simulink model "Multi_agent_MIMO"  (R2022b)
settings: Solver=VariableStepAuto  StartTime=0.0  StopTime=10.0  RelTol=1e-3
undefined symbols (not defined in the file): Angular, Linear
libraries: robotlib x9
settings Model: Creator=yoav  LastModifiedBy=yoav

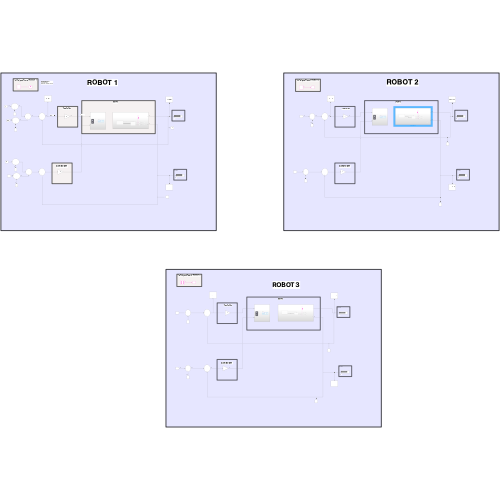
[thumbnail: Simulink's stored preview of the top-level diagram]
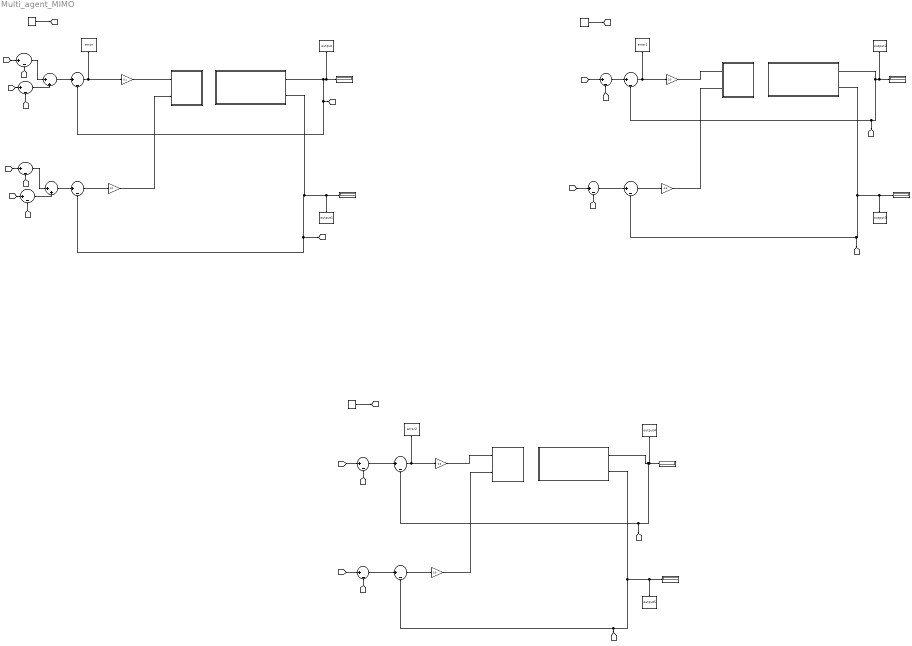
== system Multi_agent_MIMO ==
  note: The user need to
      |  put the initial position
      |  of the robot as it
      |  apperas in the spawn service
  note: $V_{command}(t)$
  note: Error - $e(t)$
  note: X
  note: Position
  note: ROBOT 2
  note: Controller
  note: Controller
  note: Controller
  note: Y
  note: Plant
  note: Position
  note: Plant
  note: Position
  note: X
  note: Controller
  note: Y
  note: Position
  note: Y
  note: Controller
  note: Position
  note: Plant
  note: X
  note: Position
  note: Controller
  note: ROBOT 1
  note: ROBOT 3
  note: Initial position of ROBOT 1
  note: Initial position of ROBOT 2
  note: Initial position of ROBOT 3
  Constant1 : Constant  Value="[5 ;  8]"  VectorParams1D=off
  Constant2 : Constant  Value="[2 ;  -4]"  VectorParams1D=off
  Constant6 : Constant  Value="[-6 ;  2]"  VectorParams1D=off
  Display{1..6} (6 alike) : Display
  Gain1 : Gain  Gain=0.1
  Gain2 : Gain  Gain=0.1
  Gain{3..6} (4 alike) : Gain  Gain=0.5
  Subsystem : Subsystem
  Subsystem1 : Subsystem
  Subsystem2 : Subsystem
  Subsystem3 : Subsystem
  Subsystem4 : Subsystem
  Subsystem5 : Subsystem
  Sum{,1..5,7..8,10..15} (14 alike) : Sum  Inputs=|+-
  Sum6 : Sum  Inputs=|++
  Sum9 : Sum  Inputs=|++
  To Workspace : ToWorkspace  VariableName=error  SaveFormat=Timeseries  SampleTime=-1
  To Workspace1 : ToWorkspace  VariableName=output  SaveFormat=Timeseries  SampleTime=-1
  To Workspace2 : ToWorkspace  VariableName=output1  SaveFormat=Timeseries  SampleTime=-1
  To Workspace3 : ToWorkspace  VariableName=error1  SaveFormat=Timeseries  SampleTime=-1
  To Workspace4 : ToWorkspace  VariableName=output2  SaveFormat=Timeseries  SampleTime=-1
  To Workspace5 : ToWorkspace  VariableName=output3  SaveFormat=Timeseries  SampleTime=-1
  To Workspace6 : ToWorkspace  VariableName=error2  SaveFormat=Timeseries  SampleTime=-1
  To Workspace7 : ToWorkspace  VariableName=output4  SaveFormat=Timeseries  SampleTime=-1
  To Workspace8 : ToWorkspace  VariableName=output5  SaveFormat=Timeseries  SampleTime=-1
  tag scope: IC1=global, IC2=global, IC3=global
  wires:
  Sum12/1 -> Sum2/1
  [Y2] -> Sum13/2
  Subsystem1/1(Output) -> Sum/2, [X1], Display3/1, To Workspace1/1
  [Y1] -> Sum10/2
  Sum5/1 -> Gain6/1
  [X3] -> Sum14/2
  Gain4/1 -> Subsystem2/2(In2)
  Gain5/1 -> Subsystem4/1(In1)
  Subsystem3/1(Output) -> [X2], Sum2/2, Display4/1, To Workspace4/1
  [X1] -> Sum14/1
  [Y1] -> Sum15/1
  Sum7/1 -> Sum6/1
  Sum9/1 -> Sum1/1
  Sum8/1 -> Sum6/2
  Sum14/1 -> Sum4/1
  Sum10/1 -> Sum9/1
  [X2] -> Sum12/2
  [Y3] -> Sum15/2
  Gain2/1 -> Subsystem/2(In2)
  Sum/1 -> To Workspace/1, Gain1/1
  Sum6/1 -> Sum/1
  Subsystem1/2(Out1) -> Sum1/2, [Y1], Display1/1, To Workspace2/1
  Subsystem3/2(Out1) -> [Y2], Sum3/2, Display2/1, To Workspace5/1
  [Y1] -> Sum11/2
  [Y2] -> Sum10/1
  Sum1/1 -> Gain2/1
  Gain3/1 -> Subsystem2/1(In1)
  [X2] -> Sum7/1
  Sum2/1 -> To Workspace3/1, Gain3/1
  Sum13/1 -> Sum3/1
  Sum15/1 -> Sum5/1
  Sum3/1 -> Gain4/1
  Sum4/1 -> To Workspace6/1, Gain5/1
  Sum11/1 -> Sum9/2
  Gain6/1 -> Subsystem4/2(In2)
  [X1] -> Sum12/1
  [X1] -> Sum7/2
  [X3] -> Sum8/1
  [Y3] -> Sum11/1
  Subsystem5/2(Out1) -> Sum5/2, [Y3], Display5/1, To Workspace8/1
  [X1] -> Sum8/2
  Subsystem5/1(Output) -> Sum4/2, [X3], Display6/1, To Workspace7/1
  Gain1/1 -> Subsystem/1(In1)
  [Y1] -> Sum13/1
  Constant6/1 -> [IC1]
  Constant1/1 -> [IC2]
  Constant2/1 -> [IC3]

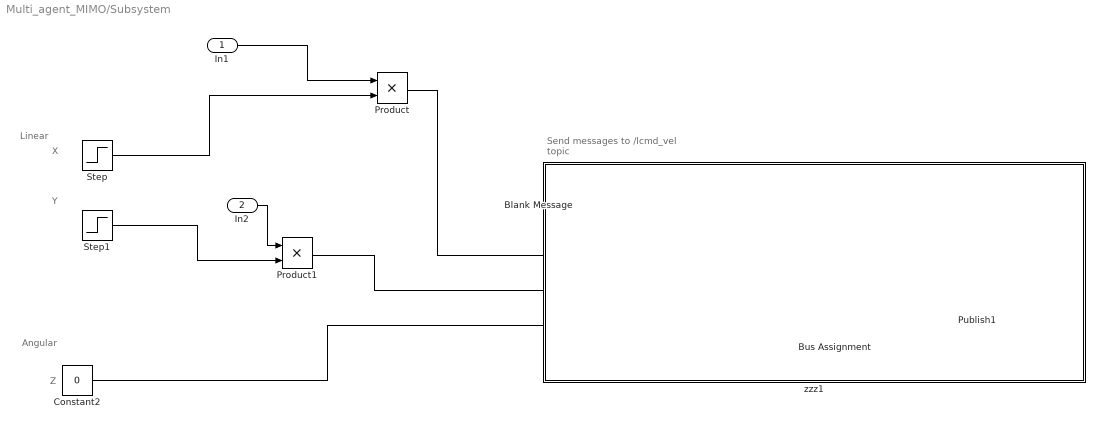
== system Multi_agent_MIMO/Subsystem ==
  note: Send messages to /lcmd_vel topic
  note: Y
  note: X
  note: Linear
  note: Angular
  note: Z
  In1 : Inport
  In2 : Inport  Port=2
  Blank Message : robotlib/Blank Message  messageClass=Message  entityType=geometry_msgs/Twist  messageType=geometry_msgs/Twist  SampleTime=inf  legacyBusStruct=off
  Bus Assignment : BusAssignment  AssignedSignals=Linear.X,Linear.Y,Angular.Z
  Constant2 : Constant  Value=0
  Product : Product
  Product1 : Product
  Publish1 : robotlib/Publish  topicSource=Specify your own  topic=/robot1/cmd_vel  messageType=geometry_msgs/Twist  legacyBusStruct=off  messageQueueLength=105
  Step : Step  Time=0  SampleTime=0
  Step1 : Step  Time=0  SampleTime=0
  zzz1 : Subsystem  TreatAsAtomicUnit=on
      settings: OpenFcn=% no-op
      mask Display: disp('')
  wires:
  Blank Message/1 -> Bus Assignment/1
  Bus Assignment/1 -> Publish1/1
  Constant2/1 -> Bus Assignment/4
  In1/1 -> Product/1
  Step/1 -> Product/2
  Product/1 -> Bus Assignment/2
  Step1/1 -> Product1/2
  In2/1 -> Product1/1
  Product1/1 -> Bus Assignment/3

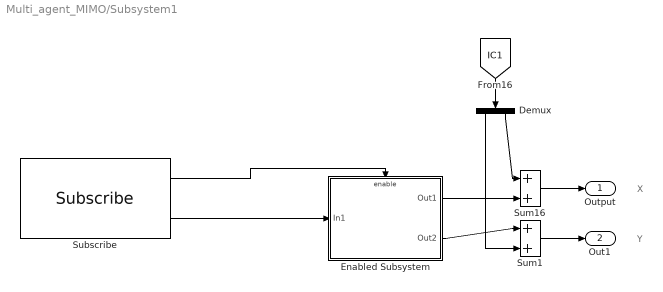
== system Multi_agent_MIMO/Subsystem1 ==
  note: X
  note: Y
  Demux : Demux  Outputs=2
  Enabled Subsystem : Subsystem  TreatAsAtomicUnit=on
  Subscribe : robotlib/Subscribe  topicSource=Select from ROS network  topic=/robot1/odom  messageType=nav_msgs/Odometry  SampleTime=-1  legacyBusStruct=off  messageQueueLength=1
      settings: LibrarySourceBlock=roslib/ROS/Subscribe
  Sum1 : Sum  Inputs=|++
  Sum16 : Sum  Inputs=|++
  Output : Outport
  Out1 : Outport  Port=2
  wires:
  Subscribe/2 -> Enabled Subsystem/1(In1)
  Subscribe/1 -> Enabled Subsystem/Enable
  Enabled Subsystem/1(Out1) -> Sum16/2
  [IC1] -> Demux/1
  Demux/2 -> Sum16/1
  Sum16/1 -> Output/1
  Enabled Subsystem/2(Out2) -> Sum1/1
  Demux/1 -> Sum1/2
  Sum1/1 -> Out1/1

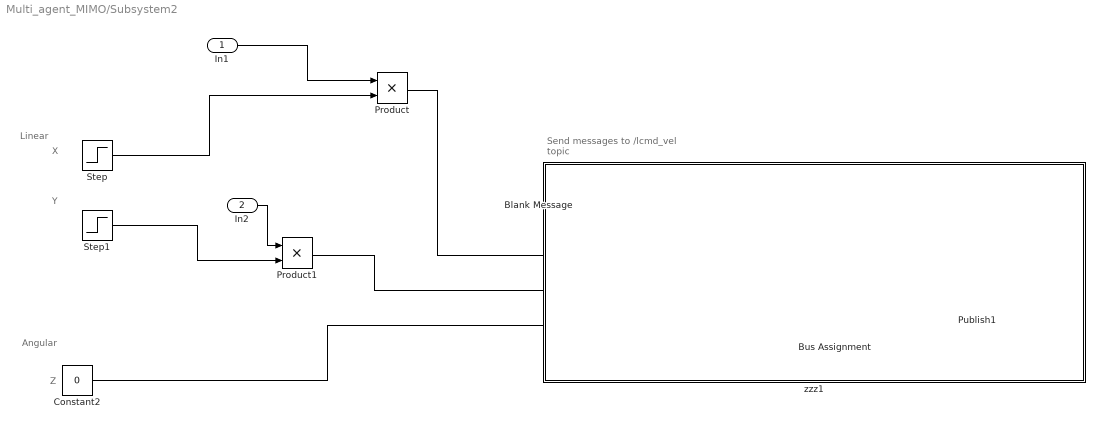
== system Multi_agent_MIMO/Subsystem2 ==
  note: Send messages to /lcmd_vel topic
  note: Y
  note: X
  note: Linear
  note: Angular
  note: Z
  In1 : Inport
  In2 : Inport  Port=2
  Blank Message : robotlib/Blank Message  messageClass=Message  entityType=geometry_msgs/Twist  messageType=geometry_msgs/Twist  SampleTime=inf  legacyBusStruct=off
  Bus Assignment : BusAssignment  AssignedSignals=Linear.X,Linear.Y,Angular.Z
  Constant2 : Constant  Value=0
  Product : Product
  Product1 : Product
  Publish1 : robotlib/Publish  topicSource=Specify your own  topic=/robot2/cmd_vel  messageType=geometry_msgs/Twist  legacyBusStruct=off  messageQueueLength=105
  Step : Step  Time=0  SampleTime=0
  Step1 : Step  Time=0  SampleTime=0
  zzz1 : Subsystem  TreatAsAtomicUnit=on
      settings: OpenFcn=% no-op
      mask Display: disp('')
  wires:
  Blank Message/1 -> Bus Assignment/1
  Bus Assignment/1 -> Publish1/1
  Constant2/1 -> Bus Assignment/4
  In1/1 -> Product/1
  Step/1 -> Product/2
  Product/1 -> Bus Assignment/2
  Step1/1 -> Product1/2
  In2/1 -> Product1/1
  Product1/1 -> Bus Assignment/3

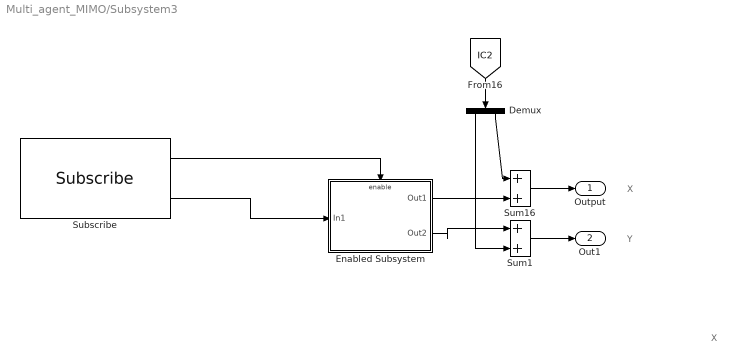
== system Multi_agent_MIMO/Subsystem3 ==
  note: X
  note: Y
  note: X
  Demux : Demux  Outputs=2
  Enabled Subsystem : Subsystem  TreatAsAtomicUnit=on
  Subscribe : robotlib/Subscribe  topicSource=Select from ROS network  topic=/robot2/odom  messageType=nav_msgs/Odometry  SampleTime=-1  legacyBusStruct=off  messageQueueLength=1
      settings: LibrarySourceBlock=roslib/ROS/Subscribe
  Sum1 : Sum  Inputs=|++
  Sum16 : Sum  Inputs=|++
  Output : Outport
  Out1 : Outport  Port=2
  wires:
  Subscribe/2 -> Enabled Subsystem/1(In1)
  Subscribe/1 -> Enabled Subsystem/Enable
  Enabled Subsystem/2(Out2) -> Sum1/1
  Demux/2 -> Sum16/1
  Enabled Subsystem/1(Out1) -> Sum16/2
  Demux/1 -> Sum1/2
  Sum1/1 -> Out1/1
  Sum16/1 -> Output/1
  [IC2] -> Demux/1

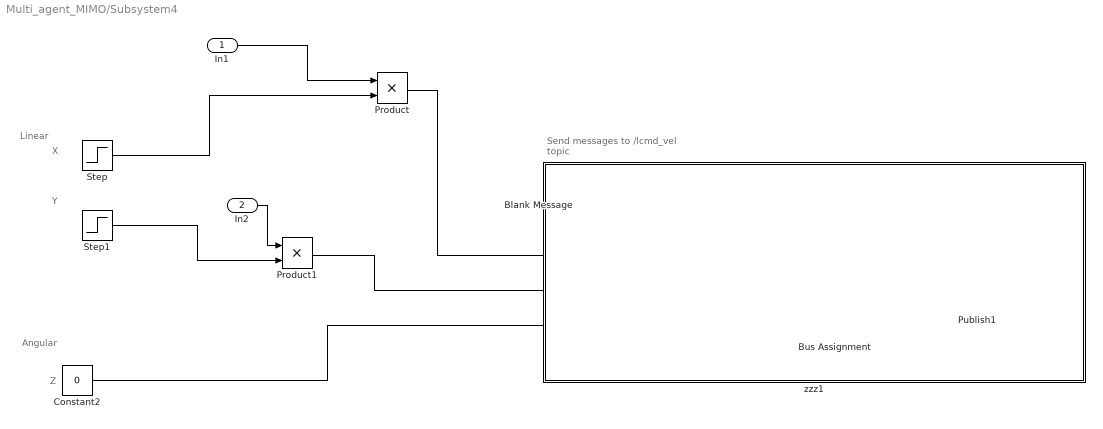
== system Multi_agent_MIMO/Subsystem4 ==
  note: Send messages to /lcmd_vel topic
  note: Y
  note: X
  note: Linear
  note: Angular
  note: Z
  In1 : Inport
  In2 : Inport  Port=2
  Blank Message : robotlib/Blank Message  messageClass=Message  entityType=geometry_msgs/Twist  messageType=geometry_msgs/Twist  SampleTime=inf  legacyBusStruct=off
  Bus Assignment : BusAssignment  AssignedSignals=Linear.X,Linear.Y,Angular.Z
  Constant2 : Constant  Value=0
  Product : Product
  Product1 : Product
  Publish1 : robotlib/Publish  topicSource=Specify your own  topic=/robot3/cmd_vel  messageType=geometry_msgs/Twist  legacyBusStruct=off  messageQueueLength=105
  Step : Step  Time=0  SampleTime=0
  Step1 : Step  Time=0  SampleTime=0
  zzz1 : Subsystem  TreatAsAtomicUnit=on
      settings: OpenFcn=% no-op
      mask Display: disp('')
  wires:
  Blank Message/1 -> Bus Assignment/1
  Bus Assignment/1 -> Publish1/1
  Constant2/1 -> Bus Assignment/4
  In1/1 -> Product/1
  Step/1 -> Product/2
  Product/1 -> Bus Assignment/2
  Step1/1 -> Product1/2
  In2/1 -> Product1/1
  Product1/1 -> Bus Assignment/3

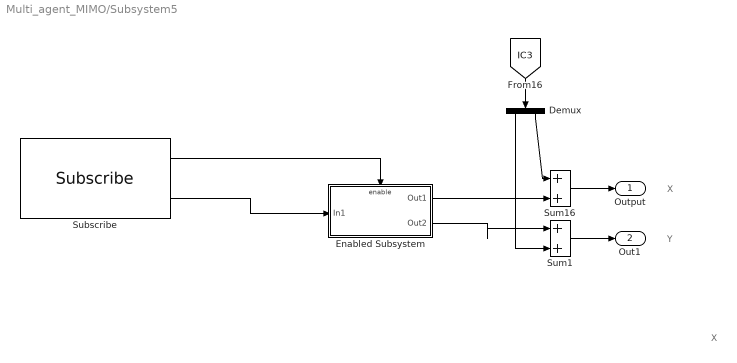
== system Multi_agent_MIMO/Subsystem5 ==
  note: X
  note: X
  note: Y
  Demux : Demux  Outputs=2
  Enabled Subsystem : Subsystem  TreatAsAtomicUnit=on
  Subscribe : robotlib/Subscribe  topicSource=Select from ROS network  topic=/robot3/odom  messageType=nav_msgs/Odometry  SampleTime=-1  legacyBusStruct=off  messageQueueLength=1
      settings: LibrarySourceBlock=roslib/ROS/Subscribe
  Sum1 : Sum  Inputs=|++
  Sum16 : Sum  Inputs=|++
  Output : Outport
  Out1 : Outport  Port=2
  wires:
  Subscribe/2 -> Enabled Subsystem/1(In1)
  Subscribe/1 -> Enabled Subsystem/Enable
  Enabled Subsystem/1(Out1) -> Sum16/2
  [IC3] -> Demux/1
  Sum16/1 -> Output/1
  Demux/1 -> Sum1/2
  Demux/2 -> Sum16/1
  Sum1/1 -> Out1/1
  Enabled Subsystem/2(Out2) -> Sum1/1

== system Multi_agent_MIMO/Subsystem/zzz1 ==

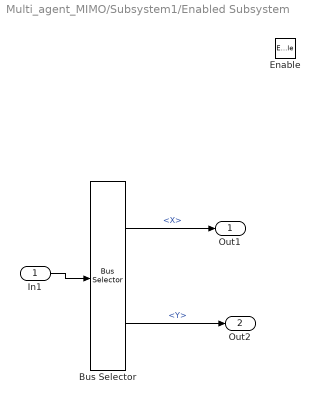
== system Multi_agent_MIMO/Subsystem1/Enabled Subsystem ==
  In1 : Inport
  Enable : EnablePort
  Bus Selector : BusSelector  OutputSignals=Pose.Pose.Position.X,Pose.Pose.Position.Y
  Out1 : Outport
  Out2 : Outport  Port=2
  wires:
  In1/1 -> Bus Selector/1
  Bus Selector/1 -> Out1/1  "<X>"
  Bus Selector/2 -> Out2/1  "<Y>"

== system Multi_agent_MIMO/Subsystem2/zzz1 ==

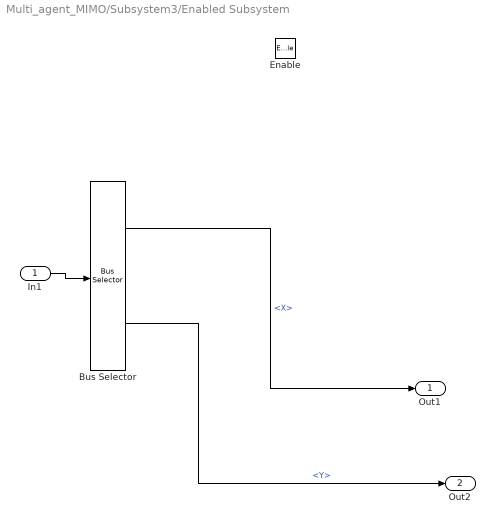
== system Multi_agent_MIMO/Subsystem3/Enabled Subsystem ==
  In1 : Inport
  Enable : EnablePort
  Bus Selector : BusSelector  OutputSignals=Pose.Pose.Position.X,Pose.Pose.Position.Y
  Out1 : Outport
  Out2 : Outport  Port=2
  wires:
  In1/1 -> Bus Selector/1
  Bus Selector/1 -> Out1/1  "<X>"
  Bus Selector/2 -> Out2/1  "<Y>"

== system Multi_agent_MIMO/Subsystem4/zzz1 ==

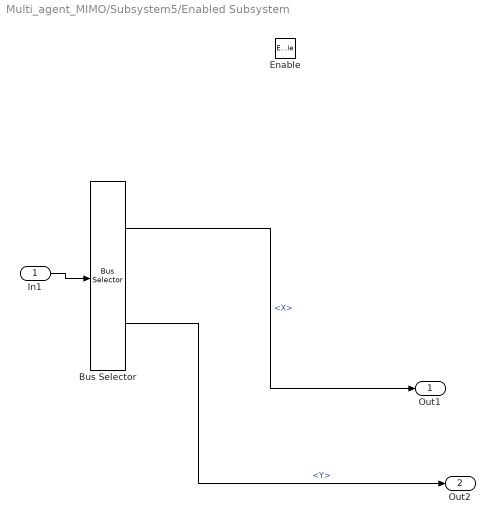
== system Multi_agent_MIMO/Subsystem5/Enabled Subsystem ==
  In1 : Inport
  Enable : EnablePort
  Bus Selector : BusSelector  OutputSignals=Pose.Pose.Position.X,Pose.Pose.Position.Y
  Out1 : Outport
  Out2 : Outport  Port=2
  wires:
  In1/1 -> Bus Selector/1
  Bus Selector/1 -> Out1/1  "<X>"
  Bus Selector/2 -> Out2/1  "<Y>"
